simulink model "Modelo_MV_CIGRE_IPSD"  (R2019b)
settings: Solver=FixedStepAuto  StartTime=0.0  StopTime=0.3  FixedStep=Ts  RelTol=1e-3
PreLoadFcn:
  | r_1=0.501
  | l_1=0.716/(60*2*pi)
  | c_1=10e-6/(60*2*pi)
  | r_0=0.817
  | l_0=1.598 /(60*2*pi)
  | c_0=10e-6/(60*2*pi)
  | Sb=50e6
  | Ts=1e-4
InitFcn:
  | r_1=0.501;
  | l_1=0.716/(60*2*pi);
  | c_1=10e-6/(60*2*pi);
  | r_0=0.817;
  | l_0=1.598 /(60*2*pi);
  | c_0=10e-6/(60*2*pi);
  | Sb=50e6;
  | Ts=1e-4;
StartFcn:
  | r_1=0.501
  | l_1=0.716/(60*2*pi)
  | c_1=10e-6/(60*2*pi)
  | r_0=0.817
  | l_0=1.598 /(60*2*pi)
  | c_0=10e-6/(60*2*pi)
  | Sb=50e6
  | Ts=1e-5
undefined symbols (not defined in the file): D1, Delta
libraries: powerlib_meascontrol x112, powerlib x55, simulink x6
(part 3 of 3)

== matlab function Modelo_MV_CIGRE_IPSD/Bus PCC/Optim_OP2 ==
  data: y1 input; y2 input; y3 input; y4 input; tout output; flag input; ag_type input; ext input
function tout = optim_operacion(y1,y2,y3,y4,flag, ag_type,ext)
    CTI=0.1;
    yt=[y1 y2 y3 y4];
    tout=ones(1,length(yt))*10000;  
    p=0;
    if flag>0 %%se verifica que se mantengan las condiciones de falla
        top=ones(1,length(yt))*10000;        
        A=zeros(length(yt),length(yt));
        C=zeros(length(yt),length(yt));
        for i=1:length(A) %creación de matrices de coordinación
            if yt(i)==1
                p=i; % se guarda donde se encuentra una falla adelante (solo para eventos unicos)
                C(i,i)=yt(i); 
            else % se crea matriz de coordinación
                A(i,i)=yt(i);
                C(i,i)=yt(i);
            end                
        end
        if p~=0
            for i=1:length(A)
                if A(i,i)==-1
                    A(i,p)=1;
                end
            end
        end
        
        j=1;
        B=ones(rank(A),length(yt));
        for i=1:length(A) %extracción de equipos de respaldo
            if A(i,i)==-1
                B(j,:)=A(i,:);
                j=j+1;
            end
        end
        h=2;
        if p==0     % No hay equipo primario al interior del bus
            if rank(C)==0
            else
                for i=1:length(yt) %Falla en la barra
                    if yt(i)==-1
                        top(1,i)=0.04;
                    end
                end
            end
        else
        switch ag_type(p)
            case 1
               top(1,p)=0.04;
            case 2
                top(1,p)=0.04;
            case 3 
                if or(yt(p)*ext(p)==1,yt(p)*ext(p)==0)
                    top(1,p)=0.04;
                else
                    top(1,p)=10000;
                end
            otherwise
                top(1,p)=10000;
        end
        
        while h~=1
            for i=1:length(yt)
                if yt(i)==-1
                    top(1,i)=top(1,p)+0.3;
                end
            end
            Rest=B*top';
            if Rest<=-CTI
                h=1;
            else
                h=2;
            end
        end
        end
    else
        top=ones(1,length(yt))*10000;
    end
    tout=top;
end

== matlab function Modelo_MV_CIGRE_IPSD/Bus10_UA/Carga 2 ==
  data: V input; y output; I input; Th_v input; Th_i input; Th_r input; I_pf input
function y = Prot_Carga(V,I,Th_v,Th_i,Th_r,I_pf)
    ag=2;
    Vth=0.9;
    Ith=1.1;
    if or(V<Vth)
        Th_rf=Th_v-Th_i;
        if abs(Th_rf-Th_r)<2
            y=0; %%No falla
        else
            if or(Th_rf>=90,Th_rf<=-90)
                y=-1; %%Falla atras
            else
                y=1; %%Falla adelante
            end
        end
    else
        y=0; %% No falla
    end
end

== matlab function Modelo_MV_CIGRE_IPSD/Bus PCC/MATLAB Function1 ==
  data: V input; Th_r output; I input; Th_v input; Th_i input; Th_r input; I_r input; I_r output
function [Th_r,I_r] = Calc_Ang(V,I,Th_v,Th_i,Th_r,I_r)
    Ith=1.1;
    Vth=0.99;
    if or(and(I<Ith,V>=Vth),V>=Vth)
        Th_r=Th_v-Th_i;
        I_r=I;
    else
        Th_r=Th_r;
        I_r=I_r;
    end
end

== matlab function Modelo_MV_CIGRE_IPSD/Bus DER/Carga 4 ==
  data: V input; y output; I input; Th_v input; Th_i input; Th_r input; ag output; I_pf input
function [y,ag] = Prot_Carga(V,I,Th_v,Th_i,Th_r,I_pf)
    ag=3;
    Vth=0.9;
    Ith=1.1;
    if or(and(I>Ith,V<Vth),and(V<Vth,I_pf-I<0))
        Th_rf=Th_v-Th_i;
        if abs(Th_rf-Th_r)<5
            y=0; %%No falla
        else
            if or(Th_rf>=90,Th_rf<=-90)
                y=-1; %%Falla atras
            else
                y=1; %%Falla adelante
            end
        end
    else
        y=0; %% No falla
    end
end

== matlab function Modelo_MV_CIGRE_IPSD/Bus DER/MATLAB Function4 ==
  data: V input; Th_r output; I input; Th_v input; Th_i input; Th_r input; I_r input; I_r output
function [Th_r,I_r] = Calc_Ang(V,I,Th_v,Th_i,Th_r,I_r)
    Ith=1.1;
    Vth=0.99;
    if or(and(I<Ith,V>=Vth),V>=Vth)
        Th_r=Th_v-Th_i;
        I_r=I;
    else
        Th_r=Th_r;
        I_r=I_r;
    end
end

== matlab function Modelo_MV_CIGRE_IPSD/Bus DER/Optim_OP2 ==
  data: y1 input; y2 input; y3 input; y4 input; y5 input; tout output; flag input; ag_type input; ext input
function tout = optim_operacion(y1,y2,y3,y4,y5,flag, ag_type,ext)
    CTI=0.1;
    yt=[y1 y2 y3 y4 y5];
    tout=ones(1,length(yt))*10000;  
    p=0;
    if flag>0 %%se verifica que se mantengan las condiciones de falla
        top=ones(1,length(yt))*10000;        
        A=zeros(length(yt),length(yt));
        C=zeros(length(yt),length(yt));
        for i=1:length(A) %creación de matrices de coordinación
            if yt(i)==1
                p=i; % se guarda donde se encuentra una falla adelante (solo para eventos unicos)
                C(i,i)=yt(i); 
            else % se crea matriz de coordinación
                A(i,i)=yt(i);
                C(i,i)=yt(i);
            end                
        end
        if p~=0
            for i=1:length(A)
                if A(i,i)==-1
                    A(i,p)=1;
                end
            end
        end
        
        j=1;
        B=ones(rank(A),length(yt));
        for i=1:length(A) %extracción de equipos de respaldo
            if A(i,i)==-1
                B(j,:)=A(i,:);
                j=j+1;
            end
        end
        h=2;
        if p==0     % No hay equipo primario al interior del bus
            if rank(C)==0
            else
                for i=1:length(yt) %Falla en la barra
                    if yt(i)==-1
                        top(1,i)=0.04;
                    end
                end
            end
        else
        switch ag_type(p)
            case 1
               top(1,p)=0.04;
            case 2
                top(1,p)=0.04;
            case 3 
                if or(yt(p)*ext(p)==1,yt(p)*ext(p)==0)
                    top(1,p)=0.04;
                else
                    top(1,p)=10000;
                end
            otherwise
                top(1,p)=10000;
        end
        
        while h~=1
            for i=1:length(yt)
                if yt(i)==-1
                    top(1,i)=top(1,p)+0.3;
                end
            end
            Rest=B*top';
            if Rest<=-CTI
                h=1;
            else
                h=2;
            end
        end
        end
    else
        top=ones(1,length(yt))*10000;
    end
    tout=top;
end

== matlab function Modelo_MV_CIGRE_IPSD/Bus PCC/Carga 4 ==
  data: V input; y output; I input; Th_v input; Th_i input; Th_r input; ag output; I_pf input
function [y,ag] = Prot_Carga(V,I,Th_v,Th_i,Th_r,I_pf)
    ag=3;
    Vth=0.9;
    Ith=1.1;
    if or(and(I>Ith,V<Vth),and(V<Vth,I_pf-I<0))
        Th_rf=Th_v-Th_i;
        if abs(Th_rf-Th_r)<5
            y=0; %%No falla
        else
            if or(Th_rf>=90,Th_rf<=-90)
                y=-1; %%Falla atras
            else
                y=1; %%Falla adelante
            end
        end
    else
        y=0; %% No falla
    end
end

== matlab function Modelo_MV_CIGRE_IPSD/Bus PCC/MATLAB Function3 ==
  data: V input; Th_r output; I input; Th_v input; Th_i input; Th_r input; I_r input; I_r output
function [Th_r,I_r] = Calc_Ang(V,I,Th_v,Th_i,Th_r,I_r)
    Ith=1.1;
    Vth=0.99;
    if or(and(I<Ith,V>=Vth),V>=Vth)
        Th_r=Th_v-Th_i;
        I_r=I;
    else
        Th_r=Th_r;
        I_r=I_r;
    end
end

== matlab function Modelo_MV_CIGRE_IPSD/Bus8_UA/MATLAB Function ==
  data: AG input; top output; Rlloc input; Rnloc input; tnop input; ext input; extl output
function [top,extl] = optim1(AG,Rlloc,Rnloc,tnop,ext)
CTI=0.3;
top=100000;
extl=3;
p=0;
if (and(or(AG==1,AG==2),Rlloc~=0)) %Load or Generator Agents
    if Rlloc==1 %Primary Operation
        top=0.01;
    elseif Rlloc==-1 %Backup Operation
        A=zeros(length(Rnloc)+1,length(Rnloc)+1);
        for i=1:length(A)
            if i==1
                A(i,i)=Rlloc;
            else
                if Rnloc(i-1)==1
                    p=i;
                end
                A(i,i)=Rnloc(i-1);
            end
        end
        for i=1:length(A)
            if A(i,i)==-1
                A(i,p)=A(p,p);
            end
        end
        h=2;
        while h~=1 %Distributed Optimization problem
            top=tnop(p-1)+0.3;
            if (tnop(p-1)-top)<=-CTI
                h=1;
            end
        end                       
    end
elseif AG==3 %Line Agent
    
    if Rlloc==1
        extl=1; %Primary operation transmited
        if ext==1
            top=0.01; %Primary operation mode
        elseif ext==0
            top=0.31; %Remote backup operation
        else
            top=100000; %Block operation
        end
    elseif Rlloc==-1
        t=0;
        for i=1:length(Rnloc)
            if Rnloc(i)==1
                t=t+1;
            end
        end
        if t==0
            top=0.01; %Primary operation mode
            extl=0;   %Inside fault transmition
        else %Local backup operation mode
            extl=2;   %Local operation transmition
            A=zeros(length(Rnloc)+1,length(Rnloc)+1);
            for i=1:length(A)
                if i==1
                    A(i,i)=Rlloc;
                else
                    if Rnloc(i-1)==1
                        p=i;
                    end
                    A(i,i)=Rnloc(i-1);
                end

            end
            for i=1:length(A)
                if A(i,i)==-1
                    A(i,p)=A(p,p);
                end
            end
            h=2;
            while h~=1 %Optimization problem
                top=tnop(p-1)+0.3;
                if (tnop(p-1)-top)<=-CTI
                    h=1;
                end
            end                       
        end
    end
end
end

== matlab function Modelo_MV_CIGRE_IPSD/Bus8_UA/Carga 2 ==
  data: V input; y output; I input; Th_v input; Th_i input; Th_r input; I_pf input
function y = Prot_Carga(V,I,Th_v,Th_i,Th_r,I_pf)
    ag=2;
    Vth=0.9;
    Ith=1.1;
    if or(V<Vth)
        Th_rf=Th_v-Th_i;
        if abs(Th_rf-Th_r)<2
            y=0; %%No falla
        else
            if or(Th_rf>=90,Th_rf<=-90)
                y=-1; %%Falla atras
            else
                y=1; %%Falla adelante
            end
        end
    else
        y=0; %% No falla
    end
end

== matlab function Modelo_MV_CIGRE_IPSD/Bus11_UA/Carga 2 ==
  data: V input; y output; I input; Th_v input; Th_i input; Th_r input; I_pf input
function y = Prot_Carga(V,I,Th_v,Th_i,Th_r,I_pf)
    ag=2;
    Vth=0.9;
    Ith=1.1;
    if or(V<Vth)
        Th_rf=Th_v-Th_i;
        if abs(Th_rf-Th_r)<2
            y=0; %%No falla
        else
            if or(Th_rf>=90,Th_rf<=-90)
                y=-1; %%Falla atras
            else
                y=1; %%Falla adelante
            end
        end
    else
        y=0; %% No falla
    end
end

== matlab function Modelo_MV_CIGRE_IPSD/Bus10_UA/MATLAB Function1 ==
  data: V input; Th_r output; I input; Th_v input; Th_i input; Th_r input; I_r input; I_r output
function [Th_r,I_r] = Calc_Ang(V,I,Th_v,Th_i,Th_r,I_r)
    Ith=1.1;
    Vth=0.99;
    if or(and(I<Ith,V>=Vth),V>=Vth)
        Th_r=Th_v-Th_i;
        I_r=I;
    else
        Th_r=Th_r;
        I_r=I_r;
    end
end

== matlab function Modelo_MV_CIGRE_IPSD/Bus8_UA/MATLAB Function1 ==
  data: V input; Th_r output; I input; Th_v input; Th_i input; Th_r input; I_r input; I_r output
function [Th_r,I_r] = Calc_Ang(V,I,Th_v,Th_i,Th_r,I_r)
    Ith=1.1;
    Vth=0.99;
    if or(and(I<Ith,V>=Vth),V>=Vth)
        Th_r=Th_v-Th_i;
        I_r=I;
    else
        Th_r=Th_r;
        I_r=I_r;
    end
end

== matlab function Modelo_MV_CIGRE_IPSD/Bus10_UA/MATLAB Function ==
  data: AG input; top output; Rlloc input; Rnloc input; tnop input; ext input; extl output
function [top,extl] = optim1(AG,Rlloc,Rnloc,tnop,ext)
CTI=0.3;
top=100000;
extl=3;
p=0;
if (and(or(AG==1,AG==2),Rlloc~=0)) %Load or Generator Agents
    if Rlloc==1 %Primary Operation
        top=0.01;
    elseif Rlloc==-1 %Backup Operation
        A=zeros(length(Rnloc)+1,length(Rnloc)+1);
        for i=1:length(A)
            if i==1
                A(i,i)=Rlloc;
            else
                if Rnloc(i-1)==1
                    p=i;
                end
                A(i,i)=Rnloc(i-1);
            end
        end
        for i=1:length(A)
            if A(i,i)==-1
                A(i,p)=A(p,p);
            end
        end
        h=2;
        while h~=1 %Distributed Optimization problem
            top=tnop(p-1)+0.3;
            if (tnop(p-1)-top)<=-CTI
                h=1;
            end
        end                       
    end
elseif AG==3 %Line Agent
    
    if Rlloc==1
        extl=1; %Primary operation transmited
        if ext==1
            top=0.01; %Primary operation mode
        elseif ext==0
            top=0.31; %Remote backup operation
        else
            top=100000; %Block operation
        end
    elseif Rlloc==-1
        t=0;
        for i=1:length(Rnloc)
            if Rnloc(i)==1
                t=t+1;
            end
        end
        if t==0
            top=0.01; %Primary operation mode
            extl=0;   %Inside fault transmition
        else %Local backup operation mode
            extl=2;   %Local operation transmition
            A=zeros(length(Rnloc)+1,length(Rnloc)+1);
            for i=1:length(A)
                if i==1
                    A(i,i)=Rlloc;
                else
                    if Rnloc(i-1)==1
                        p=i;
                    end
                    A(i,i)=Rnloc(i-1);
                end

            end
            for i=1:length(A)
                if A(i,i)==-1
                    A(i,p)=A(p,p);
                end
            end
            h=2;
            while h~=1 %Optimization problem
                top=tnop(p-1)+0.3;
                if (tnop(p-1)-top)<=-CTI
                    h=1;
                end
            end                       
        end
    end
end
end

== matlab function Modelo_MV_CIGRE_IPSD/Bus14_UA/Carga 2 ==
  data: V input; y output; I input; Th_v input; Th_i input; Th_r input; I_pf input
function y = Prot_Carga(V,I,Th_v,Th_i,Th_r,I_pf)
    ag=2;
    Vth=0.9;
    Ith=1.1;
    if (V<Vth)
        Th_rf=Th_v-Th_i;
        if abs(Th_rf-Th_r)<2
            y=0; %%No falla
        else
            if or(Th_rf>=90,Th_rf<=-90)
                y=-1; %%Falla atras
            else
                y=1; %%Falla adelante
            end
        end
    else
        y=0; %% No falla
    end
end

== matlab function Modelo_MV_CIGRE_IPSD/Bus11_UA/MATLAB Function ==
  data: AG input; top output; Rlloc input; Rnloc input; tnop input; ext input; extl output
function [top,extl] = optim1(AG,Rlloc,Rnloc,tnop,ext)
CTI=0.3;
top=100000;
extl=3;
p=0;
if (and(or(AG==1,AG==2),Rlloc~=0)) %Load or Generator Agents
    if Rlloc==1 %Primary Operation
        top=0.01;
    elseif Rlloc==-1 %Backup Operation
        A=zeros(length(Rnloc)+1,length(Rnloc)+1);
        for i=1:length(A)
            if i==1
                A(i,i)=Rlloc;
            else
                if Rnloc(i-1)==1
                    p=i;
                end
                A(i,i)=Rnloc(i-1);
            end
        end
        for i=1:length(A)
            if A(i,i)==-1
                A(i,p)=A(p,p);
            end
        end
        h=2;
        while h~=1 %Distributed Optimization problem
            top=tnop(p-1)+0.3;
            if (tnop(p-1)-top)<=-CTI
                h=1;
            end
        end                       
    end
elseif AG==3 %Line Agent
    
    if Rlloc==1
        extl=1; %Primary operation transmited
        if ext==1
            top=0.01; %Primary operation mode
        elseif ext==0
            top=0.31; %Remote backup operation
        else
            top=100000; %Block operation
        end
    elseif Rlloc==-1
        t=0;
        for i=1:length(Rnloc)
            if Rnloc(i)==1
                t=t+1;
            end
        end
        if t==0
            top=0.01; %Primary operation mode
            extl=0;   %Inside fault transmition
        else %Local backup operation mode
            extl=2;   %Local operation transmition
            A=zeros(length(Rnloc)+1,length(Rnloc)+1);
            for i=1:length(A)
                if i==1
                    A(i,i)=Rlloc;
                else
                    if Rnloc(i-1)==1
                        p=i;
                    end
                    A(i,i)=Rnloc(i-1);
                end

            end
            for i=1:length(A)
                if A(i,i)==-1
                    A(i,p)=A(p,p);
                end
            end
            h=2;
            while h~=1 %Optimization problem
                top=tnop(p-1)+0.3;
                if (tnop(p-1)-top)<=-CTI
                    h=1;
                end
            end                       
        end
    end
end
end

== matlab function Modelo_MV_CIGRE_IPSD/Bus11_UA/MATLAB Function1 ==
  data: V input; Th_r output; I input; Th_v input; Th_i input; Th_r input; I_r input; I_r output
function [Th_r,I_r] = Calc_Ang(V,I,Th_v,Th_i,Th_r,I_r)
    Ith=1.1;
    Vth=0.99;
    if or(and(I<Ith,V>=Vth),V>=Vth)
        Th_r=Th_v-Th_i;
        I_r=I;
    else
        Th_r=Th_r;
        I_r=I_r;
    end
end

== matlab function Modelo_MV_CIGRE_IPSD/Bus4_UA/Carga 2 ==
  data: V input; y output; I input; Th_v input; Th_i input; Th_r input; I_pf input
function y = Prot_Carga(V,I,Th_v,Th_i,Th_r,I_pf)
    ag=2;
    Vth=0.9;
    Ith=1.1;
    if or(V<Vth)
        Th_rf=Th_v-Th_i;
        if abs(Th_rf-Th_r)<2
            y=0; %%No falla
        else
            if or(Th_rf>=90,Th_rf<=-90)
                y=-1; %%Falla atras
            else
                y=1; %%Falla adelante
            end
        end
    else
        y=0; %% No falla
    end
end

== matlab function Modelo_MV_CIGRE_IPSD/Bus14_UA/MATLAB Function ==
  data: AG input; top output; Rlloc input; Rnloc input; tnop input; ext input; extl output
function [top,extl] = optim1(AG,Rlloc,Rnloc,tnop,ext)
CTI=0.3;
top=100000;
extl=3;
p=0;
if (and(or(AG==1,AG==2),Rlloc~=0)) %Load or Generator Agents
    if Rlloc==1 %Primary Operation
        top=0.01;
    elseif Rlloc==-1 %Backup Operation
        A=zeros(length(Rnloc)+1,length(Rnloc)+1);
        for i=1:length(A)
            if i==1
                A(i,i)=Rlloc;
            else
                if Rnloc(i-1)==1
                    p=i;
                end
                A(i,i)=Rnloc(i-1);
            end
        end
        for i=1:length(A)
            if A(i,i)==-1
                A(i,p)=A(p,p);
            end
        end
        h=2;
        while h~=1 %Distributed Optimization problem
            top=tnop(p-1)+0.3;
            if (tnop(p-1)-top)<=-CTI
                h=1;
            end
        end                       
    end
elseif AG==3 %Line Agent
    
    if Rlloc==1
        extl=1; %Primary operation transmited
        if ext==1
            top=0.01; %Primary operation mode
        elseif ext==0
            top=0.31; %Remote backup operation
        else
            top=100000; %Block operation
        end
    elseif Rlloc==-1
        t=0;
        for i=1:length(Rnloc)
            if Rnloc(i)==1
                t=t+1;
            end
        end
        if t==0
            top=0.01; %Primary operation mode
            extl=0;   %Inside fault transmition
        else %Local backup operation mode
            extl=2;   %Local operation transmition
            A=zeros(length(Rnloc)+1,length(Rnloc)+1);
            for i=1:length(A)
                if i==1
                    A(i,i)=Rlloc;
                else
                    if Rnloc(i-1)==1
                        p=i;
                    end
                    A(i,i)=Rnloc(i-1);
                end

            end
            for i=1:length(A)
                if A(i,i)==-1
                    A(i,p)=A(p,p);
                end
            end
            h=2;
            while h~=1 %Optimization problem
                top=tnop(p-1)+0.3;
                if (tnop(p-1)-top)<=-CTI
                    h=1;
                end
            end                       
        end
    end
end
end

== matlab function Modelo_MV_CIGRE_IPSD/Bus14_UA/MATLAB Function1 ==
  data: V input; Th_r output; I input; Th_v input; Th_i input; Th_r input; I_r input; I_r output
function [Th_r,I_r] = Calc_Ang(V,I,Th_v,Th_i,Th_r,I_r)
    Ith=1.1;
    Vth=0.99;
    if or(and(I<Ith,V>=Vth),V>=Vth)
        Th_r=Th_v-Th_i;
        I_r=I;
    else
        Th_r=Th_r;
        I_r=I_r;
    end
end

== matlab function Modelo_MV_CIGRE_IPSD/Bus2_UA/Carga 2 ==
  data: V input; y output; I input; Th_v input; Th_i input; Th_r input; I_pf input
function y = Prot_Carga(V,I,Th_v,Th_i,Th_r,I_pf)
    ag=2;
    Vth=0.9;
    Ith=1.1;
    if or(V<Vth)
        Th_rf=Th_v-Th_i;
        if abs(Th_rf-Th_r)<2
            y=0; %%No falla
        else
            if or(Th_rf>=90,Th_rf<=-90)
                y=-1; %%Falla atras
            else
                y=1; %%Falla adelante
            end
        end
    else
        y=0; %% No falla
    end
end

== matlab function Modelo_MV_CIGRE_IPSD/Bus9_UA/MATLAB Function ==
  data: AG input; top output; Rlloc input; Rnloc input; tnop input; ext input; extl output
function [top,extl] = optim1(AG,Rlloc,Rnloc,tnop,ext)
CTI=0.3;
top=100000;
extl=3;
p=0;
if (and(or(AG==1,AG==2),Rlloc~=0)) %Load or Generator Agents
    if Rlloc==1 %Primary Operation
        top=0.01;
    elseif Rlloc==-1 %Backup Operation
        A=zeros(length(Rnloc)+1,length(Rnloc)+1);
        for i=1:length(A)
            if i==1
                A(i,i)=Rlloc;
            else
                if Rnloc(i-1)==1
                    p=i;
                end
                A(i,i)=Rnloc(i-1);
            end
        end
        for i=1:length(A)
            if A(i,i)==-1
                A(i,p)=A(p,p);
            end
        end
        h=2;
        while h~=1 %Distributed Optimization problem
            top=tnop(p-1)+0.3;
            if (tnop(p-1)-top)<=-CTI
                h=1;
            end
        end                       
    end
elseif AG==3 %Line Agent
    
    if Rlloc==1
        extl=1; %Primary operation transmited
        if ext==1
            top=0.01; %Primary operation mode
        elseif ext==0
            top=0.31; %Remote backup operation
        else
            top=100000; %Block operation
        end
    elseif Rlloc==-1
        t=0;
        for i=1:length(Rnloc)
            if Rnloc(i)==1
                t=t+1;
            end
        end
        if t==0
            top=0.01; %Primary operation mode
            extl=0;   %Inside fault transmition
        else %Local backup operation mode
            extl=2;   %Local operation transmition
            A=zeros(length(Rnloc)+1,length(Rnloc)+1);
            for i=1:length(A)
                if i==1
                    A(i,i)=Rlloc;
                else
                    if Rnloc(i-1)==1
                        p=i;
                    end
                    A(i,i)=Rnloc(i-1);
                end

            end
            for i=1:length(A)
                if A(i,i)==-1
                    A(i,p)=A(p,p);
                end
            end
            h=2;
            while h~=1 %Optimization problem
                top=tnop(p-1)+0.3;
                if (tnop(p-1)-top)<=-CTI
                    h=1;
                end
            end                       
        end
    end
end
end

== matlab function Modelo_MV_CIGRE_IPSD/Bus9_UA/MATLAB Function1 ==
  data: V input; Th_r output; I input; Th_v input; Th_i input; Th_r input; I_r input; I_r output
function [Th_r,I_r] = Calc_Ang(V,I,Th_v,Th_i,Th_r,I_r)
    Ith=1.1;
    Vth=0.99;
    if or(and(I<Ith,V>=Vth),V>=Vth)
        Th_r=Th_v-Th_i;
        I_r=I;
    else
        Th_r=Th_r;
        I_r=I_r;
    end
end

== matlab function Modelo_MV_CIGRE_IPSD/Bus3_UA/Carga 2 ==
  data: V input; y output; I input; Th_v input; Th_i input; Th_r input; I_pf input
function y = Prot_Carga(V,I,Th_v,Th_i,Th_r,I_pf)
    ag=2;
    Vth=0.9;
    Ith=1.1;
    if or(V<Vth)
        Th_rf=Th_v-Th_i;
        if abs(Th_rf-Th_r)<2
            y=0; %%No falla
        else
            if or(Th_rf>=90,Th_rf<=-90)
                y=-1; %%Falla atras
            else
                y=1; %%Falla adelante
            end
        end
    else
        y=0; %% No falla
    end
end

== matlab function Modelo_MV_CIGRE_IPSD/Bus4_UA/MATLAB Function ==
  data: AG input; top output; Rlloc input; Rnloc input; tnop input; ext input; extl output
function [top,extl] = optim1(AG,Rlloc,Rnloc,tnop,ext)
CTI=0.3;
top=100000;
extl=3;
p=0;
if (and(or(AG==1,AG==2),Rlloc~=0)) %Load or Generator Agents
    if Rlloc==1 %Primary Operation
        top=0.01;
    elseif Rlloc==-1 %Backup Operation
        A=zeros(length(Rnloc)+1,length(Rnloc)+1);
        for i=1:length(A)
            if i==1
                A(i,i)=Rlloc;
            else
                if Rnloc(i-1)==1
                    p=i;
                end
                A(i,i)=Rnloc(i-1);
            end
        end
        for i=1:length(A)
            if A(i,i)==-1
                A(i,p)=A(p,p);
            end
        end
        h=2;
        while h~=1 %Distributed Optimization problem
            top=tnop(p-1)+0.3;
            if (tnop(p-1)-top)<=-CTI
                h=1;
            end
        end                       
    end
elseif AG==3 %Line Agent
    
    if Rlloc==1
        extl=1; %Primary operation transmited
        if ext==1
            top=0.01; %Primary operation mode
        elseif ext==0
            top=0.31; %Remote backup operation
        else
            top=100000; %Block operation
        end
    elseif Rlloc==-1
        t=0;
        for i=1:length(Rnloc)
            if Rnloc(i)==1
                t=t+1;
            end
        end
        if t==0
            top=0.01; %Primary operation mode
            extl=0;   %Inside fault transmition
        else %Local backup operation mode
            extl=2;   %Local operation transmition
            A=zeros(length(Rnloc)+1,length(Rnloc)+1);
            for i=1:length(A)
                if i==1
                    A(i,i)=Rlloc;
                else
                    if Rnloc(i-1)==1
                        p=i;
                    end
                    A(i,i)=Rnloc(i-1);
                end

            end
            for i=1:length(A)
                if A(i,i)==-1
                    A(i,p)=A(p,p);
                end
            end
            h=2;
            while h~=1 %Optimization problem
                top=tnop(p-1)+0.3;
                if (tnop(p-1)-top)<=-CTI
                    h=1;
                end
            end                       
        end
    end
end
end

== matlab function Modelo_MV_CIGRE_IPSD/Bus4_UA/MATLAB Function1 ==
  data: V input; Th_r output; I input; Th_v input; Th_i input; Th_r input; I_r input; I_r output
function [Th_r,I_r] = Calc_Ang(V,I,Th_v,Th_i,Th_r,I_r)
    Ith=1.1;
    Vth=0.99;
    if or(and(I<Ith,V>=Vth),V>=Vth)
        Th_r=Th_v-Th_i;
        I_r=I;
    else
        Th_r=Th_r;
        I_r=I_r;
    end
end

== matlab function Modelo_MV_CIGRE_IPSD/Bus15_UA/Carga 2 ==
  data: V input; y output; I input; Th_v input; Th_i input; Th_r input; I_pf input
function y = Prot_Carga(V,I,Th_v,Th_i,Th_r,I_pf)
    ag=2;
    Vth=0.9;
    Ith=1.1;
    if or(V<Vth)
        Th_rf=Th_v-Th_i;
        if abs(Th_rf-Th_r)<2
            y=0; %%No falla
        else
            if or(Th_rf>=90,Th_rf<=-90)
                y=-1; %%Falla atras
            else
                y=1; %%Falla adelante
            end
        end
    else
        y=0; %% No falla
    end
end

== matlab function Modelo_MV_CIGRE_IPSD/Bus2_UA/MATLAB Function ==
  data: AG input; top output; Rlloc input; Rnloc input; tnop input; ext input; extl output
function [top,extl] = optim1(AG,Rlloc,Rnloc,tnop,ext)
CTI=0.3;
top=100000;
extl=3;
p=0;
if (and(or(AG==1,AG==2),Rlloc~=0)) %Load or Generator Agents
    if Rlloc==1 %Primary Operation
        top=0.01;
    elseif Rlloc==-1 %Backup Operation
        A=zeros(length(Rnloc)+1,length(Rnloc)+1);
        for i=1:length(A)
            if i==1
                A(i,i)=Rlloc;
            else
                if Rnloc(i-1)==1
                    p=i;
                end
                A(i,i)=Rnloc(i-1);
            end
        end
        for i=1:length(A)
            if A(i,i)==-1
                A(i,p)=A(p,p);
            end
        end
        h=2;
        while h~=1 %Distributed Optimization problem
            top=tnop(p-1)+0.3;
            if (tnop(p-1)-top)<=-CTI
                h=1;
            end
        end                       
    end
elseif AG==3 %Line Agent
    
    if Rlloc==1
        extl=1; %Primary operation transmited
        if ext==1
            top=0.01; %Primary operation mode
        elseif ext==0
            top=0.31; %Remote backup operation
        else
            top=100000; %Block operation
        end
    elseif Rlloc==-1
        t=0;
        for i=1:length(Rnloc)
            if Rnloc(i)==1
                t=t+1;
            end
        end
        if t==0
            top=0.01; %Primary operation mode
            extl=0;   %Inside fault transmition
        else %Local backup operation mode
            extl=2;   %Local operation transmition
            A=zeros(length(Rnloc)+1,length(Rnloc)+1);
            for i=1:length(A)
                if i==1
                    A(i,i)=Rlloc;
                else
                    if Rnloc(i-1)==1
                        p=i;
                    end
                    A(i,i)=Rnloc(i-1);
                end

            end
            for i=1:length(A)
                if A(i,i)==-1
                    A(i,p)=A(p,p);
                end
            end
            h=2;
            while h~=1 %Optimization problem
                top=tnop(p-1)+0.3;
                if (tnop(p-1)-top)<=-CTI
                    h=1;
                end
            end                       
        end
    end
end
end

== matlab function Modelo_MV_CIGRE_IPSD/Bus2_UA/MATLAB Function1 ==
  data: V input; Th_r output; I input; Th_v input; Th_i input; Th_r input; I_r input; I_r output
function [Th_r,I_r] = Calc_Ang(V,I,Th_v,Th_i,Th_r,I_r)
    Ith=1.1;
    Vth=0.99;
    if or(and(I<Ith,V>=Vth),V>=Vth)
        Th_r=Th_v-Th_i;
        I_r=I;
    else
        Th_r=Th_r;
        I_r=I_r;
    end
end

== matlab function Modelo_MV_CIGRE_IPSD/Bus3_UA/MATLAB Function ==
  data: AG input; top output; Rlloc input; Rnloc input; tnop input; ext input; extl output
function [top,extl] = optim1(AG,Rlloc,Rnloc,tnop,ext)
CTI=0.3;
top=100000;
extl=3;
p=0;
if (and(or(AG==1,AG==2),Rlloc~=0)) %Load or Generator Agents
    if Rlloc==1 %Primary Operation
        top=0.01;
    elseif Rlloc==-1 %Backup Operation
        A=zeros(length(Rnloc)+1,length(Rnloc)+1);
        for i=1:length(A)
            if i==1
                A(i,i)=Rlloc;
            else
                if Rnloc(i-1)==1
                    p=i;
                end
                A(i,i)=Rnloc(i-1);
            end
        end
        for i=1:length(A)
            if A(i,i)==-1
                A(i,p)=A(p,p);
            end
        end
        h=2;
        while h~=1 %Distributed Optimization problem
            top=tnop(p-1)+0.3;
            if (tnop(p-1)-top)<=-CTI
                h=1;
            end
        end                       
    end
elseif AG==3 %Line Agent
    
    if Rlloc==1
        extl=1; %Primary operation transmited
        if ext==1
            top=0.01; %Primary operation mode
        elseif ext==0
            top=0.31; %Remote backup operation
        else
            top=100000; %Block operation
        end
    elseif Rlloc==-1
        t=0;
        for i=1:length(Rnloc)
            if Rnloc(i)==1
                t=t+1;
            end
        end
        if t==0
            top=0.01; %Primary operation mode
            extl=0;   %Inside fault transmition
        else %Local backup operation mode
            extl=2;   %Local operation transmition
            A=zeros(length(Rnloc)+1,length(Rnloc)+1);
            for i=1:length(A)
                if i==1
                    A(i,i)=Rlloc;
                else
                    if Rnloc(i-1)==1
                        p=i;
                    end
                    A(i,i)=Rnloc(i-1);
                end

            end
            for i=1:length(A)
                if A(i,i)==-1
                    A(i,p)=A(p,p);
                end
            end
            h=2;
            while h~=1 %Optimization problem
                top=tnop(p-1)+0.3;
                if (tnop(p-1)-top)<=-CTI
                    h=1;
                end
            end                       
        end
    end
end
end

== matlab function Modelo_MV_CIGRE_IPSD/Bus3_UA/MATLAB Function1 ==
  data: V input; Th_r output; I input; Th_v input; Th_i input; Th_r input; I_r input; I_r output
function [Th_r,I_r] = Calc_Ang(V,I,Th_v,Th_i,Th_r,I_r)
    Ith=1.1;
    Vth=0.99;
    if or(and(I<Ith,V>=Vth),V>=Vth)
        Th_r=Th_v-Th_i;
        I_r=I;
    else
        Th_r=Th_r;
        I_r=I_r;
    end
end

== matlab function Modelo_MV_CIGRE_IPSD/Bus15_UA/MATLAB Function ==
  data: AG input; top output; Rlloc input; Rnloc input; tnop input; ext input; extl output
function [top,extl] = optim1(AG,Rlloc,Rnloc,tnop,ext)
CTI=0.3;
top=100000;
extl=3;
p=0;
if (and(or(AG==1,AG==2),Rlloc~=0)) %Load or Generator Agents
    if Rlloc==1 %Primary Operation
        top=0.01;
    elseif Rlloc==-1 %Backup Operation
        A=zeros(length(Rnloc)+1,length(Rnloc)+1);
        for i=1:length(A)
            if i==1
                A(i,i)=Rlloc;
            else
                if Rnloc(i-1)==1
                    p=i;
                end
                A(i,i)=Rnloc(i-1);
            end
        end
        for i=1:length(A)
            if A(i,i)==-1
                A(i,p)=A(p,p);
            end
        end
        h=2;
        while h~=1 %Distributed Optimization problem
            top=tnop(p-1)+0.3;
            if (tnop(p-1)-top)<=-CTI
                h=1;
            end
        end                       
    end
elseif AG==3 %Line Agent
    
    if Rlloc==1
        extl=1; %Primary operation transmited
        if ext==1
            top=0.01; %Primary operation mode
        elseif ext==0
            top=0.31; %Remote backup operation
        else
            top=100000; %Block operation
        end
    elseif Rlloc==-1
        t=0;
        for i=1:length(Rnloc)
            if Rnloc(i)==1
                t=t+1;
            end
        end
        if t==0
            top=0.01; %Primary operation mode
            extl=0;   %Inside fault transmition
        else %Local backup operation mode
            extl=2;   %Local operation transmition
            A=zeros(length(Rnloc)+1,length(Rnloc)+1);
            for i=1:length(A)
                if i==1
                    A(i,i)=Rlloc;
                else
                    if Rnloc(i-1)==1
                        p=i;
                    end
                    A(i,i)=Rnloc(i-1);
                end

            end
            for i=1:length(A)
                if A(i,i)==-1
                    A(i,p)=A(p,p);
                end
            end
            h=2;
            while h~=1 %Optimization problem
                top=tnop(p-1)+0.3;
                if (tnop(p-1)-top)<=-CTI
                    h=1;
                end
            end                       
        end
    end
end
end

== matlab function Modelo_MV_CIGRE_IPSD/Bus15_UA/MATLAB Function1 ==
  data: V input; Th_r output; I input; Th_v input; Th_i input; Th_r input; I_r input; I_r output
function [Th_r,I_r] = Calc_Ang(V,I,Th_v,Th_i,Th_r,I_r)
    Ith=1.1;
    Vth=0.99;
    if or(and(I<Ith,V>=Vth),V>=Vth)
        Th_r=Th_v-Th_i;
        I_r=I;
    else
        Th_r=Th_r;
        I_r=I_r;
    end
end

== stateflow chart Modelo_MV_CIGRE_IPSD/Bus8_UA/Chart ==
  state Init
  state No_estable
    out=0
    y1=0
    on after(0.02,sec):
    y1=1
  state Estable
    out=Rlloc
  state NO_estable
    out=0
    y1=0
    on after(0.03,sec):
    y1=1
  (default) -> Init
  Init -> No_estable [order 1] : [Rlloc==1]
  No_estable -> Estable : [y1==1]
  Init -> NO_estable [order 2] : [Rlloc==-1]
  NO_estable -> Estable : [y1==1]
  data: out output double; y1 local double; Rlloc input

== stateflow chart Modelo_MV_CIGRE_IPSD/Bus9_UA/Chart ==
  state Init
  state No_estable
    out=0
    y1=0
    on after(0.02,sec):
    y1=1
  state Estable
    out=Rlloc
  state NO_estable
    out=0
    y1=0
    on after(0.03,sec):
    y1=1
  (default) -> Init
  Init -> No_estable [order 1] : [Rlloc==1]
  No_estable -> Estable : [y1==1]
  Init -> NO_estable [order 2] : [Rlloc==-1]
  NO_estable -> Estable : [y1==1]
  data: out output double; y1 local double; Rlloc input

== stateflow chart Modelo_MV_CIGRE_IPSD/Bus10_UA/Chart ==
  state Init
  state No_estable
    out=0
    y1=0
    on after(0.02,sec):
    y1=1
  state Estable
    out=Rlloc
  state NO_estable
    out=0
    y1=0
    on after(0.03,sec):
    y1=1
  (default) -> Init
  Init -> No_estable [order 1] : [Rlloc==1]
  No_estable -> Estable : [y1==1]
  Init -> NO_estable [order 2] : [Rlloc==-1]
  NO_estable -> Estable : [y1==1]
  data: out output double; y1 local double; Rlloc input

== stateflow chart Modelo_MV_CIGRE_IPSD/Bus11_UA/Chart ==
  state Init
  state No_estable
    out=0
    y1=0
    on after(0.02,sec):
    y1=1
  state Estable
    out=Rlloc
  state NO_estable
    out=0
    y1=0
    on after(0.03,sec):
    y1=1
  (default) -> Init
  Init -> No_estable [order 1] : [Rlloc==1]
  No_estable -> Estable : [y1==1]
  Init -> NO_estable [order 2] : [Rlloc==-1]
  NO_estable -> Estable : [y1==1]
  data: out output double; y1 local double; Rlloc input

== stateflow chart Modelo_MV_CIGRE_IPSD/Bus14_UA/Chart ==
  state Init
  state No_estable
    out=0
    y1=0
    on after(0.02,sec):
    y1=1
  state Estable
    out=Rlloc
  state NO_estable
    out=0
    y1=0
    on after(0.03,sec):
    y1=1
  (default) -> Init
  Init -> No_estable [order 1] : [Rlloc==1]
  No_estable -> Estable : [y1==1]
  Init -> NO_estable [order 2] : [Rlloc==-1]
  NO_estable -> Estable : [y1==1]
  data: out output double; y1 local double; Rlloc input

== stateflow chart Modelo_MV_CIGRE_IPSD/Bus4_UA/Chart ==
  state Init
  state No_estable
    out=0
    y1=0
    on after(0.02,sec):
    y1=1
  state Estable
    out=Rlloc
  state NO_estable
    out=0
    y1=0
    on after(0.03,sec):
    y1=1
  (default) -> Init
  Init -> No_estable [order 1] : [Rlloc==1]
  No_estable -> Estable : [y1==1]
  Init -> NO_estable [order 2] : [Rlloc==-1]
  NO_estable -> Estable : [y1==1]
  data: out output double; y1 local double; Rlloc input

== stateflow chart Modelo_MV_CIGRE_IPSD/Bus2_UA/Chart ==
  state Init
  state No_estable
    out=0
    y1=0
    on after(0.02,sec):
    y1=1
  state Estable
    out=Rlloc
  state NO_estable
    out=0
    y1=0
    on after(0.03,sec):
    y1=1
  (default) -> Init
  Init -> No_estable [order 1] : [Rlloc==1]
  No_estable -> Estable : [y1==1]
  Init -> NO_estable [order 2] : [Rlloc==-1]
  NO_estable -> Estable : [y1==1]
  data: out output double; y1 local double; Rlloc input

== stateflow chart Modelo_MV_CIGRE_IPSD/Bus3_UA/Chart ==
  state Init
  state No_estable
    out=0
    y1=0
    on after(0.02,sec):
    y1=1
  state Estable
    out=Rlloc
  state NO_estable
    out=0
    y1=0
    on after(0.03,sec):
    y1=1
  (default) -> Init
  Init -> No_estable [order 1] : [Rlloc==1]
  No_estable -> Estable : [y1==1]
  Init -> NO_estable [order 2] : [Rlloc==-1]
  NO_estable -> Estable : [y1==1]
  data: out output double; y1 local double; Rlloc input

== stateflow chart Modelo_MV_CIGRE_IPSD/Bus15_UA/Chart ==
  state Init
  state No_estable
    out=0
    y1=0
    on after(0.02,sec):
    y1=1
  state Estable
    out=Rlloc
  state NO_estable
    out=0
    y1=0
    on after(0.03,sec):
    y1=1
  (default) -> Init
  Init -> No_estable [order 1] : [Rlloc==1]
  No_estable -> Estable : [y1==1]
  Init -> NO_estable [order 2] : [Rlloc==-1]
  NO_estable -> Estable : [y1==1]
  data: out output double; y1 local double; Rlloc input
